simulink model "Bounce"  (R2018a)
settings: Solver=VariableStepAuto  StartTime=0.0  StopTime=10.0  RelTol=1e-3
values from neighbouring files (symbols this model uses):
  Ab = [0 1 0 0 ... (first row only)    [Bounce_controll.m]
  Bb = [0 0 0 0 ... (first row only)    [Bounce_controll.m]
  Cb = [1 0 0 0 ... (first row only)    [Bounce_controll.m]
  Db = [0 0 0 0 ... (first row only)    [Bounce_controll.m]
  sinfreq = testHZ*2*pi    (= 6.28318530718)    [Bounce_controll.m]
settings Model: Creator=c_s  LastModifiedBy=c_s

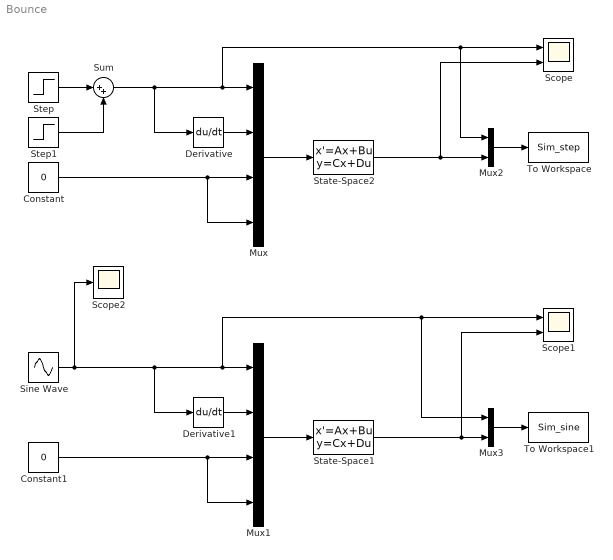
== system Bounce ==
  Constant : Constant  Value=0
  Constant1 : Constant  Value=0
  Derivative : Derivative
  Derivative1 : Derivative
  Mux : Mux
  Mux1 : Mux
  Mux2 : Mux  Inputs=2
  Mux3 : Mux  Inputs=2
  Scope : Scope  NumInputPorts=2
  Scope1 : Scope  NumInputPorts=2
  Scope2 : Scope
  Sine Wave : Sin  Amplitude=0.01  Frequency=sinfreq  SampleTime=0
  State-Space1 : StateSpace  A=Ab  B=Bb  C=Cb  D=Db  InitialCondition=0
  State-Space2 : StateSpace  A=Ab  B=Bb  C=Cb  D=Db  InitialCondition=0
  Step : Step  Time=0  After=0.03  SampleTime=0
  Step1 : Step  After=-0.03  SampleTime=0
  Sum : Sum  Inputs=|++
  To Workspace : ToWorkspace  VariableName=Sim_step  SaveFormat=Structure With Time  SampleTime=-1
  To Workspace1 : ToWorkspace  VariableName=Sim_sine  SaveFormat=Structure With Time  SampleTime=-1
  wires:
  Step1/1 -> Sum/2
  Step/1 -> Sum/1
  Mux/1 -> State-Space2/1
  Sum/1 -> Derivative/1, Mux2/1, Scope/1, Mux/1
  Constant/1 -> Mux/4, Mux/3
  Derivative/1 -> Mux/2
  Mux1/1 -> State-Space1/1
  Constant1/1 -> Mux1/4, Mux1/3
  Derivative1/1 -> Mux1/2
  Sine Wave/1 -> Scope2/1, Derivative1/1, Scope1/1, Mux3/1, Mux1/1
  Mux2/1 -> To Workspace/1
  Mux3/1 -> To Workspace1/1
  State-Space2/1 -> Scope/2, Mux2/2
  State-Space1/1 -> Scope1/2, Mux3/2
